simulink model "PowerSplitHEV"  (R2026a)
settings: Solver=VariableStepAuto  StopTime=20  MaxStep=0.2  EnableMultiTasking=on
PreLoadFcn:
  | v0                 = 15; % Initial vehicle speed
  | wheel_radius = 0.3; % Wheel radius
  | rpm0             = 2000; % Engine initial speed demand
  | ratio = 2; % Power split gear ratio
libraries: fl_lib x49, nesl_utility x16, ee_lib x3, batteryecm_lib x1
(part 2 of 2)

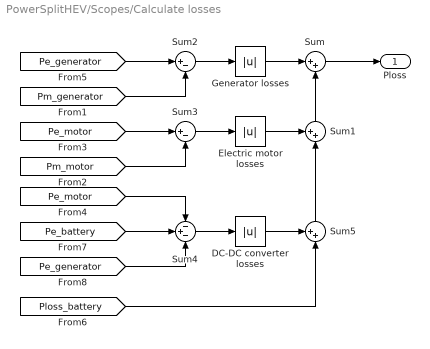
== system PowerSplitHEV/Scopes/Calculate losses ==
  " Electric motor losses" : Abs
  DC-DC converter losses : Abs
  Generator losses : Abs
  Sum : Sum  Inputs=|++
  Sum1 : Sum  Inputs=++|
  Sum2 : Sum  Inputs=|+-
  Sum3 : Sum  Inputs=|+-
  Sum4 : Sum  Inputs=-+-
  Sum5 : Sum  Inputs=++|
  Ploss : Outport  VectorParamsAs1DForOutWhenUnconnected=off
  wires:
  Sum1/1 -> Sum/2
  Sum/1 -> Ploss/1
  [Pe_generator] -> Sum2/1
  [Pm_generator] -> Sum2/2
  Sum2/1 -> Generator losses/1
  Generator losses/1 -> Sum/1
  [Pe_motor] -> Sum3/1
  [Pm_motor] -> Sum3/2
  Sum3/1 -> " Electric motor losses"/1
  Sum4/1 -> DC-DC converter losses/1
  Sum5/1 -> Sum1/2
  [Pe_battery] -> Sum4/2
  [Pe_motor] -> Sum4/1
  [Pe_generator] -> Sum4/3
  " Electric motor losses"/1 -> Sum1/1
  DC-DC converter losses/1 -> Sum5/1
  [Ploss_battery] -> Sum5/2
